simulink model "Problema8_2_Preditor"  (R2018b)
settings: Solver=VariableStepAuto  StartTime=0.0  StopTime=40.0  RelTol=1e-3
values from neighbouring files (symbols this model uses):
  A = [ -3 0; 1 0 ]    [Problema8_2.m]
  B = [ 1; 0]    [Problema8_2.m]
  C1 = [ 1 0 ]    [Problema8_2.m]
  C2 = [ 0 1 ]    [Problema8_2.m]
  Ca = [1 0;0 1]    [Problema8_2.m]
  Da = [0;0]    [Problema8_2.m]
  h = 0.2    [Problema8_2.m]
  L = [0 1] * inv(Wc) * (phi^2 + p1 * phi + p2 * eye(2))    [Problema8_2.m]
  Lc = ganho_dc/( C * inv(eye(2) - phi_cl ) * gama )    [Problema8_2.m]
  x0 = [ 0 0 ]'    [Problema8_2.m]
undefined symbols (not defined in the file or in its folder): t_in, t_per, v_in, v_per
settings Model: Creator=Asus  LastModifiedBy=fredericovaz
settings SFSimCC: SimUseLocalCustomCode=off
settings RTWCC: RTWUseLocalCustomCode=off
settings CodeAppCC: StateflowObjectComments=on

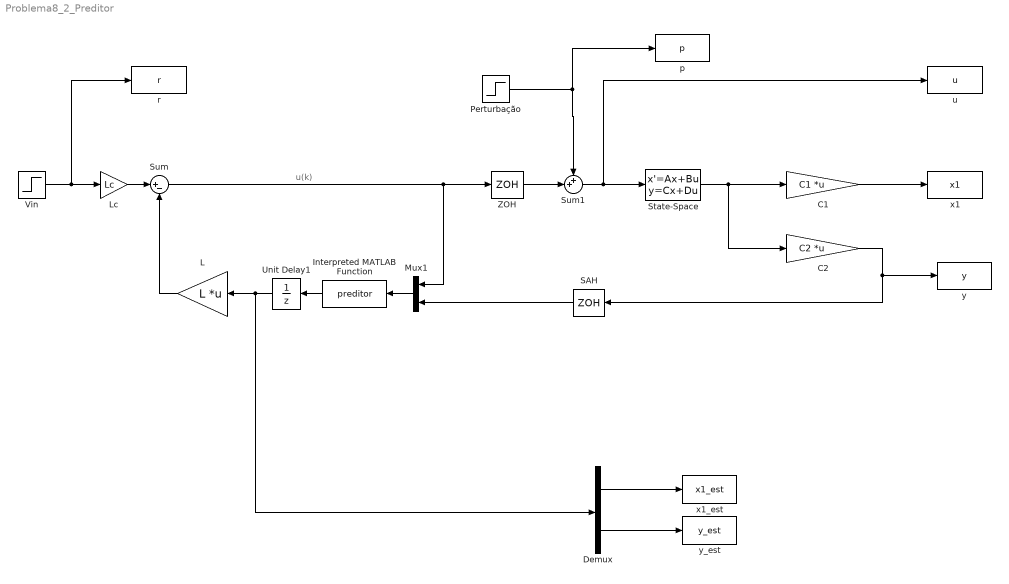
== system Problema8_2_Preditor ==
  note: u(k)
  C1 : Gain  Gain=C1  Multiplication=Matrix(K*u) (u vector)
  C2 : Gain  Gain=C2  Multiplication=Matrix(K*u) (u vector)
  Demux : Demux  Outputs=2
  Interpreted MATLAB Function : MATLABFcn  MATLABFcn=preditor  OutputDimensions=2
  L : Gain  Gain=L  Multiplication=Matrix(K*u) (u vector)
  Lc : Gain  Gain=Lc
  Mux1 : Mux  Inputs=2
  Perturbação : Step  Time=t_per  After=v_per  SampleTime=0
  SAH : ZeroOrderHold  SampleTime=h
  State-Space : StateSpace  A=A  B=B  C=Ca  D=Da  InitialCondition=x0
  Sum : Sum  Inputs=|+-
  Sum1 : Sum  Inputs=++|
  Unit Delay1 : UnitDelay  SampleTime=-1
  Vin : Step  Time=t_in  After=v_in  SampleTime=0
  ZOH : ZeroOrderHold  SampleTime=h
  p : ToWorkspace  VariableName=p  SaveFormat=Structure With Time  SampleTime=-1
  r : ToWorkspace  VariableName=r  SaveFormat=Structure With Time  SampleTime=-1
  u : ToWorkspace  VariableName=u  SaveFormat=Structure With Time  SampleTime=-1
  x1 : ToWorkspace  VariableName=x1  SaveFormat=Structure With Time  SampleTime=-1
  x1_est : ToWorkspace  VariableName=x1_est  SaveFormat=Structure With Time  SampleTime=-1
  y : ToWorkspace  VariableName=y  SaveFormat=Structure With Time  SampleTime=-1
  y_est : ToWorkspace  VariableName=y_est  SaveFormat=Structure With Time  SampleTime=-1
  wires:
  ZOH/1 -> Sum1/2
  L/1 -> Sum/2
  C2/1 -> y/1, SAH/1
  Demux/2 -> y_est/1
  Sum1/1 -> u/1, State-Space/1
  Perturbação/1 -> Sum1/1, p/1
  Lc/1 -> Sum/1
  Demux/1 -> x1_est/1
  C1/1 -> x1/1
  Vin/1 -> r/1, Lc/1
  Sum/1 -> Mux1/1, ZOH/1
  State-Space/1 -> C1/1, C2/1
  Mux1/1 -> Interpreted MATLAB Function/1
  SAH/1 -> Mux1/2
  Unit Delay1/1 -> Demux/1, L/1
  Interpreted MATLAB Function/1 -> Unit Delay1/1
